simulink model "Parallel1"  (Simulink 8.7)
settings: Solver=ode45  StartTime=0.0  StopTime=10.0  RelTol=1e-3
settings Model: Creator=scaife  LastModifiedBy=bourbouh  ExtModeAutoUpdateStatusClock=off
settings DataIOCC: SignalLoggingSaveFormat=ModelDataLogs  SignalLoggingName=sigsOut
settings DebuggingCC: SaveWithParameterizedLinksMsg=none  SignalResolutionControl=TryResolveAllWithWarning  MultiTaskDSMMsg=warning  MultiTaskCondExecSysMsg=none
settings HardwareCC: TargetUnknown=on
settings SFSimCC: SimParseCustomCode=off
settings GRTTargetCC: GeneratePreprocessorConditionals=Use local settings  CombineOutputUpdateFcns=off  GRTInterface=on

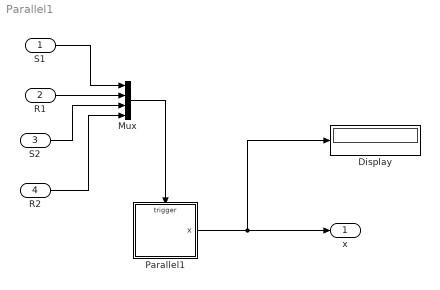
== system Parallel1 ==
  S1 : Inport
  R1 : Inport  Port=2
  S2 : Inport  Port=3
  R2 : Inport  Port=4
  Display : Display
  Mux : Mux
  Parallel1 : Stateflow chart  TreatAsAtomicUnit=on
  x : Outport
  wires:
  Parallel1/1(x) -> Display/1, x/1
  Mux/1 -> Parallel1/Trigger
  R2/1 -> Mux/4
  S2/1 -> Mux/3
  R1/1 -> Mux/2
  S1/1 -> Mux/1

== stateflow chart Parallel1 ==
  state N1/ [parallel]
    en:x+=10000;
    ex:x-=10000;
    du:x+=1000000;
    settings: executionOrder=1
    state A/
      en: x+=10;
    state B/
      en: x-=10;
    (default) -> A
    A -> B : S1
        | {x+=1;}
    B -> A : R1
        | {x-=1;}
  state N2/ [parallel]
    en:x+=100000;
    ex:x-=100000;
    settings: executionOrder=2
    state C/
      en: x+=1000;
    state D/
      en: x-=1000;
    (default) -> C
    C -> D : S2
        | {x+=100;}
    D -> C : R2
        | {x-=100;}
  data: x output int32
  events: S1 input EITHER_EDGE_EVENT; R1 input EITHER_EDGE_EVENT; S2 input EITHER_EDGE_EVENT; R2 input EITHER_EDGE_EVENT
